simulink model "Citation_2017a"  (R2017a)
settings: Solver=ode5  StartTime=0.0  StopTime=inf  FixedStep=0.01  RelTol=1e-3  EnableMultiTasking=on
InitFcn:
  | initcit
values from neighbouring files (symbols this model uses):
  aeroinit = [dp_ini;inicoef('CX0');inicoef('CXa');inicoef('CXa2');inicoef('CXq')     ;inicoef('CXde');inicoef('CY0');inicoef('CYB');inicoef('CYp');inicoef('CYr')     ;inicoef('CYda');inicoef('CYdr');inicoef('CZ0');inicoef('CZa');inicoef('CZq')     ;inicoef('CZde');inicoef('Cl0');inicoef('ClB');inicoef('Clp');inicoef('Clr')     ;inicoef('Clda');inicoef('Cldr');inicoef('Cm0');inicoef('Cma');inicoef('Cmq')     ; ...(+113 chars)    [initcit.m]
  Clda_thresh = 3.410e-2/2    (= 0.01705)    [initcit.m]
  h_l_old = zeros(6,sample_size)    [initcit.m]
  h_m_old = zeros(4,sample_size)    [initcit.m]
  h_n_old = zeros(6,sample_size)    [initcit.m]
  h_X_old = zeros(5,sample_size)    [initcit.m]
  h_Y_old = zeros(6,sample_size)    [initcit.m]
  h_Z_old = zeros(4,sample_size)    [initcit.m]
  I = [massinit(5),0, -massinit(8);0, massinit(6),0;-massinit(8),0, massinit(7)]    [initcit.m]
  p_l = [inicoef('Cl0');inicoef('ClB');inicoef('Clp');inicoef('Clr')     ;inicoef('Clda');inicoef('Cldr')].*ones(6,sample_size)    [initcit.m]
  p_m = [inicoef('Cm0');inicoef('Cma');inicoef('Cmq')     ;inicoef('Cmde')].*ones(4,sample_size)    [initcit.m]
  p_n = [inicoef('Cn0');inicoef('CnB');inicoef('Cnp');inicoef('Cnr')     ;inicoef('Cnda');inicoef('Cndr')].*ones(6,sample_size)    [initcit.m]
  p_X = [inicoef('CX0');inicoef('CXa');inicoef('CXa2');inicoef('CXq')     ;inicoef('CXde')].*ones(5,sample_size)    [initcit.m]
  p_Y = [inicoef('CY0');inicoef('CYB');inicoef('CYp');inicoef('CYr')     ;inicoef('CYda');inicoef('CYdr')].*ones(6,sample_size)    [initcit.m]
  p_Z = [inicoef('CZ0');inicoef('CZa');inicoef('CZq')     ;inicoef('CZde')].*ones(4,sample_size)    [initcit.m]
  Pcov_l = 10000*eye(6)    [initcit.m]
  Pcov_m = 10000*eye(4)    [initcit.m]
  Pcov_n = 10000*eye(6)    [initcit.m]
  Pcov_X = 10000*eye(5)    [initcit.m]
  Pcov_Y = 10000*eye(6)    [initcit.m]
  Pcov_Z = 10000*eye(4)    [initcit.m]
  replay = 0    [initcit.m]
  T0 = 288.15    [rho_test.m]
  timeend = inputsim.data{1}.Values.Time(end)    [initcit.m]
  Vw915 = 0    [initcit.m]
  winddir = 45*(pi/180)    (= 0.785398163397)    [initcit.m]
  x0 = []    [cessnac550_3d_sfnc.m]    (also in sfunxyauto.m)
  y_l = zeros(1,sample_size)    [initcit.m]
  y_l_est_old = zeros(size(y_l))    [initcit.m]
  y_m = zeros(1,sample_size)    [initcit.m]
  y_m_est_old = zeros(size(y_m))    [initcit.m]
  y_n = zeros(1,sample_size)    [initcit.m]
  y_n_est_old = zeros(size(y_n))    [initcit.m]
  y_X = zeros(1,sample_size)    [initcit.m]
  y_X_est_old = zeros(size(y_X))    [initcit.m]
  y_Y = zeros(1,sample_size)    [initcit.m]
  y_Y_est_old = zeros(size(y_Y))    [initcit.m]
  y_Z = zeros(1,sample_size)    [initcit.m]
  y_Z_est_old = zeros(size(y_Z))    [initcit.m]
undefined symbols (not defined in the file or in its folder): chord, cv1, cv2, cv3, cv4, deltagmax1, deltagmax2, deltagmax3, deltagmax4, Deng, ealphag, ealphas, g0, hDME, hGS, kt1, kt2, kt3, lh, massinit, matbuaf, matdaf, matdam, matdbbf, matdeaf, matdgaf, matdqaf, matduaf, matdwaw, matedhr, mateif, matelhr, matemhr, matemv1, matemv2, matemve, matetam, mateuaf, matfaaf, matfaxl, matff, matibaf, matibmh, matipaf, matipmh, matiraf, matiuaf, matiwaf, matlaf, matlam, matleaf, matleam, matlgaf, matlqaf, matluaf, matmaaf, matmaam, matmaf, matmam, matmbbf ... (+74)
undefined symbols (not defined in the file): matibb
libraries: simulink x13, templibrary x6, vrlib x1
(part 7 of 7)

== matlab function Citation_2017a/Pilot/Select new mode/Triggered Subsystem/MATLAB Function ==
  data: index input; triggers input; index output; triggers_pref output; triggers_pref input
function [index,triggers_pref] = fcn(index,triggers,triggers_pref)

diff=floor(triggers-triggers_pref);
triggers_pref=triggers;
nr=find(diff,1);

if not(size(find(diff,1),1)==0)
    index=nr(1);
    if index==1
        disp('Selected Control Mode: INDI')
    elseif index==2
        disp('Selected Control Mode: NDI')
    elseif index==3
        disp('Selected Control Mode: Classic rotational rate control')
    elseif index==4
        disp('Selected Control Mode: Default Actuator control')
    end
end

== matlab function Citation_2017a/Aerodynamic Parameter Estimation/alternative failure monitor system/Auto_correlation/autocorrelation ==
  data: delta input; PI_kgap output; kgap input; kgap_avg input; counter input; kgap_avg output; counter output
function [PI_kgap,kgap_avg,counter] = fcn(delta,kgap,kgap_avg,counter)

PI_kgap=(delta(1)*delta(1+kgap));
if counter>=1
    kgap_avg=kgap_avg+(PI_kgap/counter);
else
    kgap_avg=PI_kgap;
end

counter=counter+1;
end

== matlab function Citation_2017a/Aerodynamic Parameter Estimation/alternative failure monitor system/moving average square ==
  data: delta input; av output
function av = fcn(delta)
av=0;
nav=length(delta);
k=nav;
for i=0:(nav-1)
    av=av+(delta(k-i))^2;
end
av=av/k;
end

== matlab function Citation_2017a/Aerodynamic Parameter Estimation/alternative failure monitor system/variance/MATLAB Function ==
  data: delta input; var output; delta_avg input; counter input; delta_avg output; counter output; sigma_avg input; sigma_avg output
function [var,delta_avg,counter,sigma_avg] = variance(delta,delta_avg,counter,sigma_avg)

if counter >=1
    delta_avg=delta_avg+delta/counter;
    var=0;
    if counter >=2
        var=((delta-delta_avg)^2);
        
        s=sigma_avg(1)+(sqrt(var)/(counter-1));
        sigma_avg=[s;-s];
    end
else
    delta_avg=delta;
    var=0;
end



counter=counter+1;

== matlab function Citation_2017a/Aerodynamic Parameter Estimation/Statistics 2/Auto_correlation/autocorrelation ==
  data: delta input; PI_kgap output; kgap input; kgap_avg input; counter input; kgap_avg output; counter output
function [PI_kgap,kgap_avg,counter] = fcn(delta,kgap,kgap_avg,counter)

PI_kgap=(delta(1)*delta(1+kgap));
if counter>=1
    kgap_avg=kgap_avg+(PI_kgap/counter);
else
    kgap_avg=PI_kgap;
end

counter=counter+1;
end

== matlab function Citation_2017a/Aerodynamic Parameter Estimation/Statistics 2/moving average square ==
  data: delta input; av output
function av = fcn(delta)
av=0;
nav=length(delta);
k=nav;
for i=0:(nav-1)
    av=av+(delta(k-i))^2;
end
av=av/k;
end

== matlab function Citation_2017a/Aerodynamic Parameter Estimation/Statistics 2/variance/MATLAB Function ==
  data: delta input; var output; delta_avg input; counter input; delta_avg output; counter output; sigma_avg input; sigma_avg output
function [var,delta_avg,counter,sigma_avg] = variance(delta,delta_avg,counter,sigma_avg)

if counter >=1
    delta_avg=delta_avg+delta/counter;
    var=0;
    if counter >=2
        var=((delta-delta_avg)^2);
        
        s=sigma_avg(1)+sqrt(var)/(counter-1);
        sigma_avg=[s;-s];
    end
else
    delta_avg=delta;
    var=0;
end



counter=counter+1;

== matlab function Citation_2017a/Aerodynamic Parameter Estimation/Statistics 3/Auto_correlation/autocorrelation ==
  data: delta input; PI_kgap output; kgap input; kgap_avg input; counter input; kgap_avg output; counter output
function [PI_kgap,kgap_avg,counter] = fcn(delta,kgap,kgap_avg,counter)

PI_kgap=(delta(1)*delta(1+kgap));
if counter>=1
    kgap_avg=kgap_avg+(PI_kgap/counter);
else
    kgap_avg=PI_kgap;
end

counter=counter+1;
end

== matlab function Citation_2017a/Aerodynamic Parameter Estimation/Statistics 3/moving average square ==
  data: delta input; av output
function av = fcn(delta)
av=0;
nav=length(delta);
k=nav;
for i=0:(nav-1)
    av=av+(delta(k-i))^2;
end
av=av/k;
end

== matlab function Citation_2017a/Aerodynamic Parameter Estimation/Statistics 3/variance/MATLAB Function ==
  data: delta input; var output; delta_avg input; counter input; delta_avg output; counter output; sigma_avg input; sigma_avg output
function [var,delta_avg,counter,sigma_avg] = variance(delta,delta_avg,counter,sigma_avg)

if counter >=1
    delta_avg=delta_avg+delta/counter;
    var=0;
    if counter >=2
        var=((delta-delta_avg)^2);
        
        s=sigma_avg(1)+(sqrt(var)/(counter-1));
        sigma_avg=[s;-s];
    end
else
    delta_avg=delta;
    var=0;
end



counter=counter+1;

== matlab function Citation_2017a/Aerodynamic Parameter Estimation/Statistics 4/Auto_correlation/autocorrelation ==
  data: delta input; PI_kgap output; kgap input; kgap_avg input; counter input; kgap_avg output; counter output
function [PI_kgap,kgap_avg,counter] = fcn(delta,kgap,kgap_avg,counter)

PI_kgap=(delta(1)*delta(1+kgap));
if counter>=1
    kgap_avg=kgap_avg+(PI_kgap/counter);
else
    kgap_avg=PI_kgap;
end

counter=counter+1;
end

== matlab function Citation_2017a/Aerodynamic Parameter Estimation/Statistics 4/moving average square ==
  data: delta input; av output
function av = fcn(delta)
av=0;
nav=length(delta);
k=nav;
for i=0:(nav-1)
    av=av+(delta(k-i))^2;
end
av=av/k;
end

== matlab function Citation_2017a/Aerodynamic Parameter Estimation/Statistics 4/variance/MATLAB Function ==
  data: delta input; var output; delta_avg input; counter input; delta_avg output; counter output; sigma_avg input; sigma_avg output
function [var,delta_avg,counter,sigma_avg] = variance(delta,delta_avg,counter,sigma_avg)

if counter >=1
    delta_avg=delta_avg+delta/counter;
    var=0;
    if counter >=2
        var=((delta-delta_avg)^2);
        
        s=sigma_avg(1)+sqrt(var)/(counter-1);
        sigma_avg=[s;-s];
    end
else
    delta_avg=delta;
    var=0;
end



counter=counter+1;

== matlab function Citation_2017a/Pilot/button2toggle 6/MATLAB Function ==
function  fcn()

disp('PID Integral values have been reset manually');

== matlab function Citation_2017a/Aerodynamic Parameter Estimation/alternative failure monitor system/Send diagnostic message/MATLAB Function ==
  data: u input
function  fcn(u)

if u>0
    disp('Failure Detected');
else
    disp('Failure disappearance detected');
    
end

== matlab function Citation_2017a/Aerodynamic Parameter Estimation/Failure monitor system /MATLAB Function ==
  data: u input; y output double; counter input; counter output; deaf_window parameter
function [y,counter] = fcn(u,counter,deaf_window)

if counter>0
    counter=counter+1;
end

if u>0 && counter==0
    y=1;
    counter=counter+1;
else
    y=0;
end


if counter>deaf_window
    counter=0;    
end
y=y(1);

== matlab function Citation_2017a/Controllers/INDI rotational rate controller/INDI ==
  data: dp input; control_input output; e_omegadot input; I parameter; aeroinit parameter; control_input input; chord parameter; span parameter
function control_input = fcn(dp,e_omegadot,I, aeroinit, control_input,chord, span)
Clda=aeroinit(21);
Cldr=aeroinit(22);
Cmde=aeroinit(26);
Cnda=aeroinit(31);
Cndr=aeroinit(32);
mat=[span*Clda, 0, span*Cldr; 
      0,chord*Cmde,0; 
      span*Cnda, 0, span*Cndr];
  

delta_control_input=mat^(-1)*(I/dp)*e_omegadot; %delta_da; delta_de; delta_dr 
control_input=control_input+[delta_control_input(2);delta_control_input(1);delta_control_input(3)]; %this corrects the order of flight control inputs

%correct order: de; da; dr

== matlab function Citation_2017a/Controllers/ANDI rotational rate controller/a ==
  data: aerodat input; state input; y output; I parameter; span parameter; chord parameter
function y = fcn(aerodat,state, I, span, chord)
dp=aerodat(1);
p=state(1);
q=state(2);
r=state(3);
b=span;
c=chord;
V=state(4);
alpha=state(5);
beta=state(6);
Cl=aerodat(17:22);
Cm=aerodat(23:26);
Cn=aerodat(27:32);


Cla=Cl(1)+Cl(2)*beta+(Cl(3)*(p*b)/(2*V))+(Cl(4)*(r*b/(2*V)));
Cma=Cm(1)+Cm(2)*alpha+(Cm(3)*(q*c)/(2*V));
Cna=Cn(1)+Cn(2)*beta+(Cn(3)*(p*b)/(2*V))+(Cn(4)*(r*b/(2*V)));
term1=cross(state(1:3),I*state(1:3));
term2=dp*[b*Cla; c*Cma; b*Cna];
term3=term1-term2;
y=-1*(I^(-1)*term3);

== matlab function Citation_2017a/Controllers/ANDI rotational rate controller/b^-1 ==
  data: ve input; delta output; aerodat input; I parameter; chord parameter; span parameter; mat_old output; mat_old input
function [delta, mat_old]  = fcn(ve,aerodat, I, chord, span,mat_old)
dp=aerodat(1); %dynamic pressure =0.5*rho*V^2*S
clda=aerodat(21);
cldr=aerodat(22);
cmde=aerodat(26);
cnda=aerodat(31);
cndr=aerodat(32);
mat=[span*clda, 0, span*cldr;
    0, chord*cmde, 0;
    span*cnda, 0, span*cndr];

if det(mat)==0 %take an older matrix if it is non-invertible
   mat=mat_old; 
else
    mat_old=mat;
end
amat=mat^(-1)*I;
delta=amat*(1/(dp))*ve;

== matlab function Citation_2017a/Aerodynamic Parameter Estimation/Failure monitor system /Send message/MATLAB Function ==
function  fcn()

disp('Failure event detected');
end
